simulink model "projeto"  (R2023b)
settings: Solver=VariableStepAuto  StartTime=0.0  StopTime=1000  RelTol=1e-3
settings Model: Creator=natha  LastModifiedBy=natha

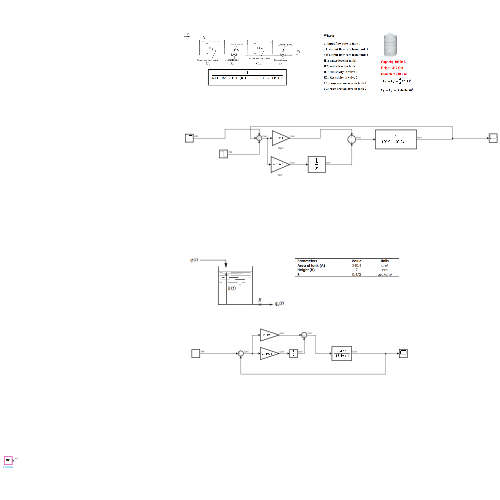
[thumbnail: Simulink's stored preview of the top-level diagram]
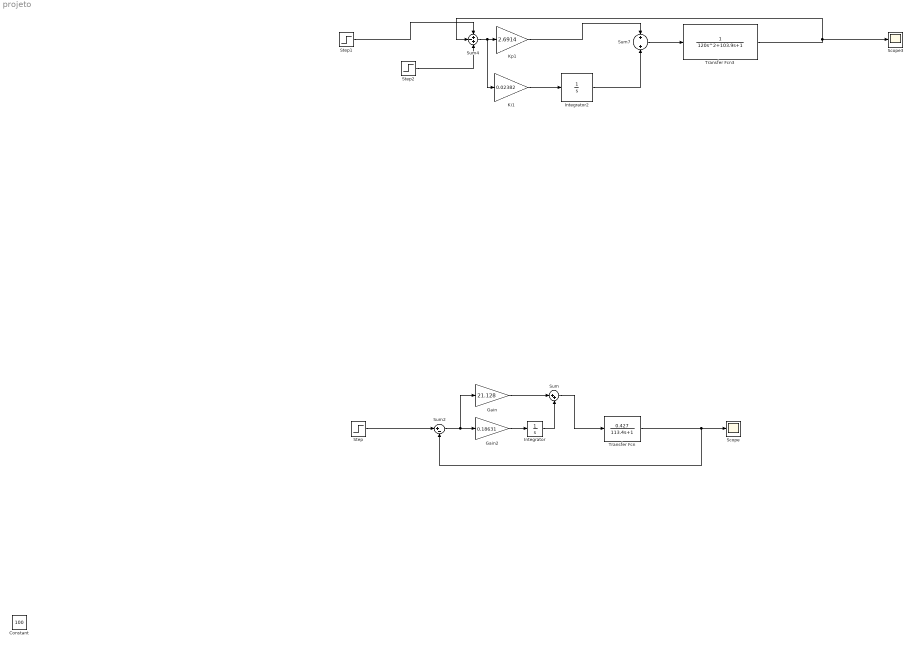
== system projeto ==
  Constant : Constant  Value=100
  Gain : Gain  Gain=21.128
  Gain2 : Gain  Gain=0.18631
  Integrator : Integrator
  Integrator2 : Integrator
  Ki1 : Gain  Gain=0.02382
  Kp1 : Gain  Gain=2.6914
  Scope : Scope
  Scope3 : Scope
  Step : Step  After=100  SampleTime=0
  Step1 : Step  After=100  SampleTime=0
  Step2 : Step  Time=300  After=-50  SampleTime=0
  Sum : Sum  Inputs=|++
  Sum2 : Sum  Inputs=|+-  SaturateOnIntegerOverflow=on
  Sum4 : Sum  Inputs=+-+  SaturateOnIntegerOverflow=on
  Sum7 : Sum
  Transfer Fcn : TransferFcn  Numerator=[0.427]  Denominator=[113.4 1]
  Transfer Fcn3 : TransferFcn  Denominator=[120 103.9 1]
  wires:
  Sum2/1 -> Gain2/1, Gain/1
  Sum/1 -> Transfer Fcn/1
  Gain/1 -> Sum/1
  Integrator/1 -> Sum/2
  Gain2/1 -> Integrator/1
  Transfer Fcn/1 -> Sum2/2, Scope/1
  Transfer Fcn3/1 -> Scope3/1, Sum4/2
  Ki1/1 -> Integrator2/1
  Integrator2/1 -> Sum7/2
  Kp1/1 -> Sum7/1
  Sum4/1 -> Ki1/1, Kp1/1
  Step/1 -> Sum2/1
  Step1/1 -> Sum4/1
  Sum7/1 -> Transfer Fcn3/1
  Step2/1 -> Sum4/3
